simulink model "CTRL_DSI_test"  (R2023b)
settings: Solver=VariableStepAuto  StartTime=0.0  StopTime=10.0  RelTol=1e-3
libraries: CTRL_DSI x1, simulink x1
settings Model: Creator=blatak  LastModifiedBy=blatak

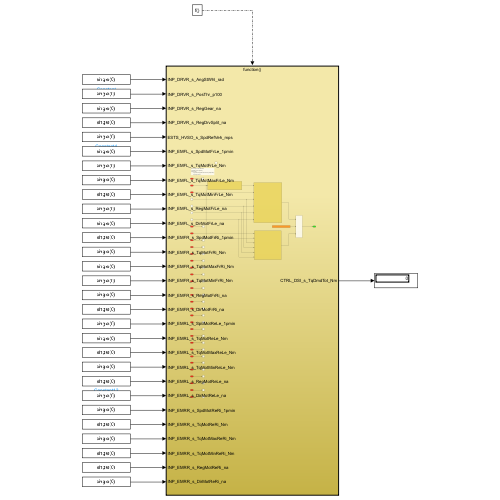
[thumbnail: Simulink's stored preview of the top-level diagram]
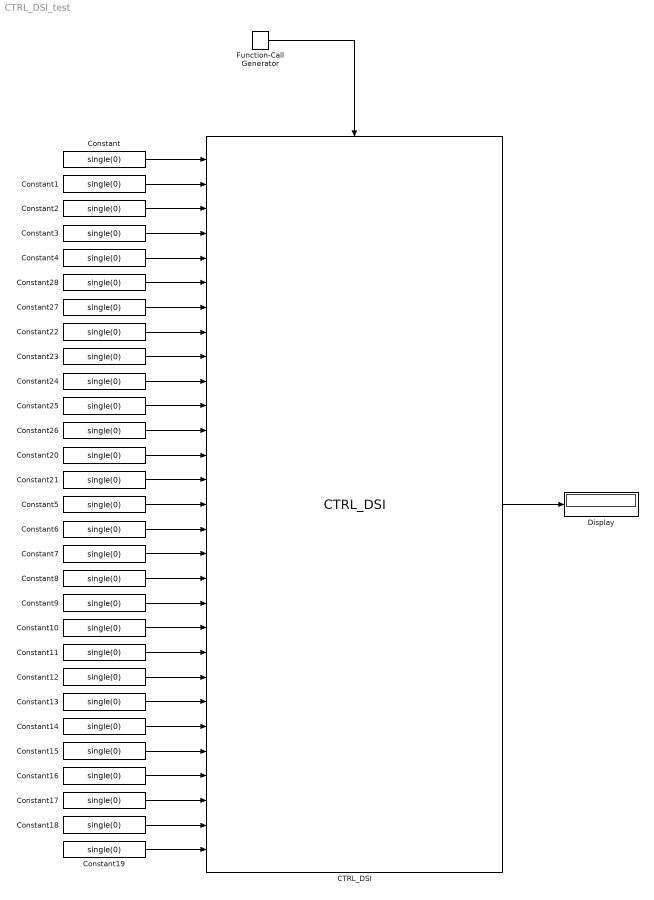
== system CTRL_DSI_test ==
  CTRL_DSI : CTRL_DSI/CTRL_DSI  SystemSampleTime=-1  VariantActivationTime=update diagram  AllowFlexibleInterface=on  Latency=0  AutoFrameSizeCalculation=off
  Constant{,1..28} (29 alike) : Constant  Value=single(0)
  Display : Display
  Function-Call Generator : simulink/Ports & Subsystems/Function-Call Generator  sample_time=0.01  numberOfIterations=1  DisallowWideOutput=off
  wires:
  Constant/1 -> CTRL_DSI/1
  Constant1/1 -> CTRL_DSI/2
  Constant2/1 -> CTRL_DSI/3
  Constant3/1 -> CTRL_DSI/4
  Constant4/1 -> CTRL_DSI/5
  Constant28/1 -> CTRL_DSI/6
  Constant27/1 -> CTRL_DSI/7
  Constant22/1 -> CTRL_DSI/8
  Constant23/1 -> CTRL_DSI/9
  Constant24/1 -> CTRL_DSI/10
  Constant25/1 -> CTRL_DSI/11
  Constant26/1 -> CTRL_DSI/12
  Constant20/1 -> CTRL_DSI/13
  Constant21/1 -> CTRL_DSI/14
  Constant5/1 -> CTRL_DSI/15
  Constant6/1 -> CTRL_DSI/16
  Constant7/1 -> CTRL_DSI/17
  Constant8/1 -> CTRL_DSI/18
  Constant9/1 -> CTRL_DSI/19
  Constant10/1 -> CTRL_DSI/20
  Constant11/1 -> CTRL_DSI/21
  Constant12/1 -> CTRL_DSI/22
  Constant13/1 -> CTRL_DSI/23
  Constant14/1 -> CTRL_DSI/24
  Constant15/1 -> CTRL_DSI/25
  Constant16/1 -> CTRL_DSI/26
  Constant17/1 -> CTRL_DSI/27
  Constant18/1 -> CTRL_DSI/28
  Constant19/1 -> CTRL_DSI/29
  CTRL_DSI/1 -> Display/1
  Function-Call Generator/1 -> CTRL_DSI/Trigger
